simulink model "statefbmodel_example_23a"  (R2023b)
settings: Solver=VariableStepAuto  StartTime=0.0  StopTime=10  RelTol=1e-6
undefined symbols (not defined in the file or in its folder): A, B, C, K
settings Model: Creator=cbirdson  LastModifiedBy=aliawolken

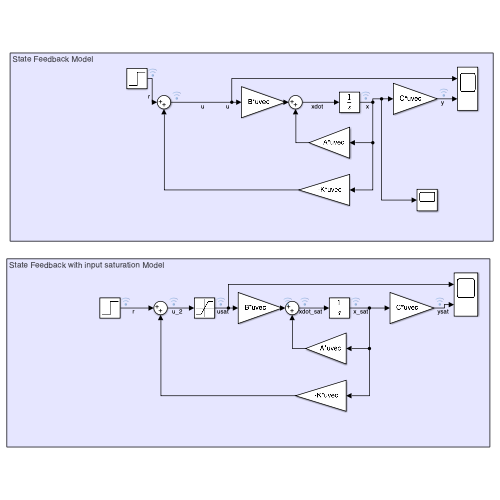
[thumbnail: Simulink's stored preview of the top-level diagram]
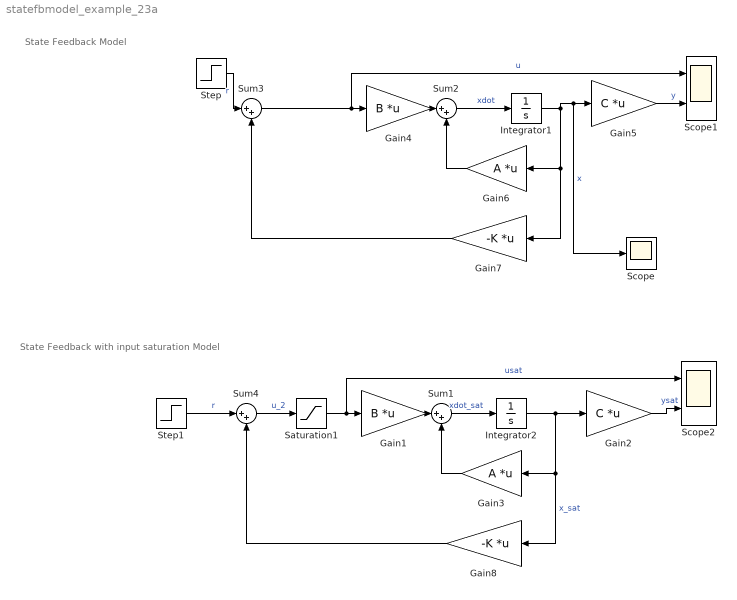
== system statefbmodel_example_23a ==
  note: State Feedback Model
  note: State Feedback with input saturation Model
  Gain1 : Gain  Gain=B  Multiplication=Matrix(K*u) (u vector)
  Gain2 : Gain  Gain=C  Multiplication=Matrix(K*u) (u vector)
  Gain3 : Gain  Gain=A  Multiplication=Matrix(K*u) (u vector)
  Gain4 : Gain  Gain=B  Multiplication=Matrix(K*u) (u vector)
  Gain5 : Gain  Gain=C  Multiplication=Matrix(K*u) (u vector)
  Gain6 : Gain  Gain=A  Multiplication=Matrix(K*u) (u vector)
  Gain7 : Gain  Gain=-K  Multiplication=Matrix(K*u) (u vector)
  Gain8 : Gain  Gain=-K  Multiplication=Matrix(K*u) (u vector)
  Integrator1 : Integrator
  Integrator2 : Integrator
  Saturation1 : Saturate  UpperLimit=1  LowerLimit=-1
  Scope : Scope
  Scope1 : Scope  NumInputPorts=2
  Scope2 : Scope  NumInputPorts=2
  Step : Step  Time=0.1  SampleTime=0
  Step1 : Step  Time=0.1  SampleTime=0
  Sum{1..4} (4 alike) : Sum  Inputs=|++
  wires:
  Gain5/1 -> Scope1/2  "y"
  Step/1 -> Sum3/1  "r"
  Gain7/1 -> Sum3/2
  Gain6/1 -> Sum2/2
  Integrator1/1 -> Scope/1, Gain5/1, Gain6/1, Gain7/1  "x"
  Sum2/1 -> Integrator1/1  "xdot"
  Gain4/1 -> Sum2/1
  Sum3/1 -> Gain4/1, Scope1/1  "u"
  Saturation1/1 -> Scope2/1, Gain1/1  "usat"
  Sum4/1 -> Saturation1/1  "u_2"
  Gain1/1 -> Sum1/1
  Sum1/1 -> Integrator2/1  "xdot_sat"
  Integrator2/1 -> Gain8/1, Gain3/1, Gain2/1  "x_sat"
  Gain3/1 -> Sum1/2
  Gain8/1 -> Sum4/2
  Step1/1 -> Sum4/1  "r"
  Gain2/1 -> Scope2/2  "ysat"
